simulink model "Balancing_Logic"  (R2024b)
settings: configuration reference "BMS_Sw_CodeGenConfig" (kept outside this file)
undefined symbols (not defined in the file): BMS_State_Enum, Ns_Module, NumModules
libraries: simulink x1, BatteryBalancing x1
settings Model: DataDictionary=DD_Balancing_Logic.sldd  ExtModeTrigDuration=5  Creator=cpatel  LastModifiedBy=97433
settings ConfigSetRef: SourceName=BMS_Sw_CodeGenConfig

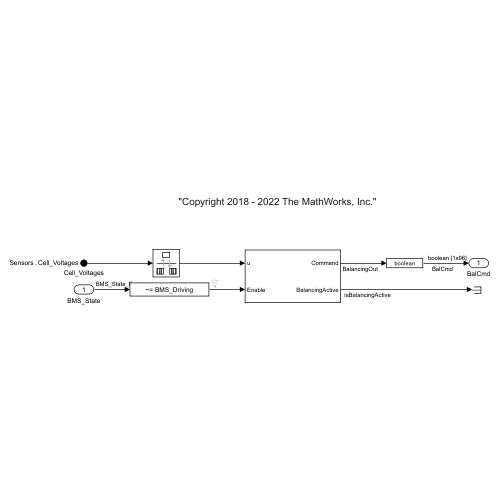
[thumbnail: Simulink's stored preview of the top-level diagram]
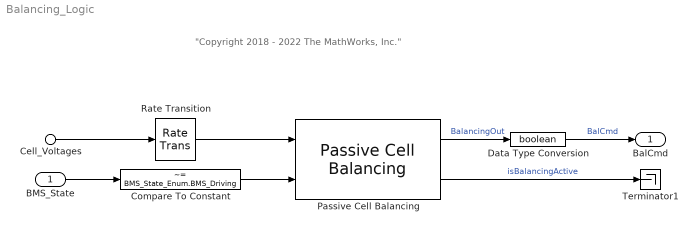
== system Balancing_Logic ==
  note: "Copyright 2018 - 2022 The MathWorks, Inc."
  BMS_State : Inport  OutDataTypeStr=Enum: BMS_State_Enum  PortDimensions=1  SampleTime=[5,0]
  Cell_Voltages : Inport  Port=2  PortName=Sensors  Element=Cell_Voltages
  Compare To Constant : simulink/Logic and Bit Operations/Compare To Constant  relop=~=  const=BMS_State_Enum.BMS_Driving  OutDataTypeStr=boolean
  Data Type Conversion : DataTypeConversion  OutDataTypeStr=boolean  SaturateOnIntegerOverflow=off  RndMeth=Floor
  Passive Cell Balancing : BatteryBalancing/Passive Cell Balancing  Threshold=0.01  HysteresisBand=0  Td_on=20  Td_off=60  Ts=5  dataType=double
      settings: LibrarySourceBlock=batt_sl_lib/Cell Balancing/Passive Cell Balancing
  Rate Transition : RateTransition  OutPortSampleTime=5
  Terminator1 : Terminator
  BalCmd : Outport  OutDataTypeStr=boolean  PortDimensions=[1,NumModules*Ns_Module]  SampleTime=[5,0]  VectorParamsAs1DForOutWhenUnconnected=off
  wires:
  BMS_State/1 -> Compare To Constant/1
  Cell_Voltages/1 -> Rate Transition/1
  Compare To Constant/1 -> Passive Cell Balancing/2
  Passive Cell Balancing/1 -> Data Type Conversion/1  "BalancingOut"
  Passive Cell Balancing/2 -> Terminator1/1  "isBalancingActive"
  Data Type Conversion/1 -> BalCmd/1  "BalCmd"
  Rate Transition/1 -> Passive Cell Balancing/1
